simulink model "FOC"  (R2015b)
settings: Solver=VariableStepAuto  StartTime=0.0  StopTime=1  FixedStep=1e-5  RelTol=1e-3
model workspace (MAT data in the model file):
  J = 0.02
  Lm = 0.651
  Lr = 0.671
  Ls = 0.666
  P = 4
  Rr = 3.24
  Rs = 4.25
  theta0 = 0
undefined symbols (not defined in the file or in its folder): magnitude
libraries: powerlib x13, simulink x3
settings Model: Creator=yoush  LastModifiedBy=yoush

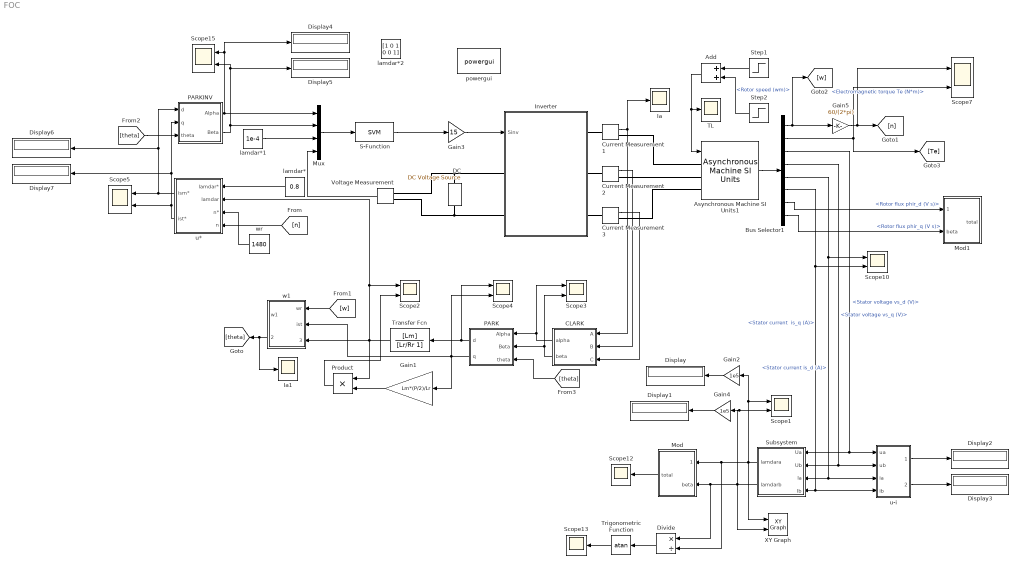
== system FOC ==
  Add : Sum
  Asynchronous Machine SI Units1 : powerlib/Machines/Asynchronous Machine SI Units  RotorType=Squirrel-cage  PresetModel=No  MechanicalLoad=Torque Tm  ShowDetailedParameters=on  ReferenceFrame=Stationary  Units=SI  MeasurementBus=off  NominalParameters=[20000 500 50]  Stator=[4.25 0.015]  Rotor=[3.24 0.020]  Cage1=[0.4155 0.002066]  Cage2=[0.4168 0.0003495]  Lm=0.651  Mechanical=[0.02 0 2]  PolePairs=2  InitialConditions=[ 1 0 0 0 0 0 0 0]  SimulateSaturation=off  Saturation=[14.03593122, 27.81365428, 53.79336849, 72.68890987, 97.98006896, 148.6815601, 215.7428561, 302.9841135, 428.7778367 ; 230, 322, 414, 460, 506, 552, 598, 644, 690]  LoadFlowParameters=1492000  TsPowergui=0  TsBlock=-1  IterativeModel=Trapezoidal non iterative  Pmec=1.492e+006
  Bus Selector1 : BusSelector  OutputSignals="Mechanical.Rotor speed (wm),Mechanical.Electromagnetic torque Te (N*m),Stator measurements.Stator voltage vs_d (V),Stator measurements.Stator voltage vs_q (V),Stator measurements.Stator current is_d (A),Stator measurements.Stator current  is_q (A),Rotor measurements.Rotor flux phir_d (V s),Rotor measurements.Rotor flux phir_q (V s)"
  CLARK : Subsystem
  Current Measurement1 : powerlib/Measurements/Current Measurement  PhasorSimulation=off  OutputType=Complex  PSBequivalent=0
  Current Measurement2 : powerlib/Measurements/Current Measurement  PhasorSimulation=off  OutputType=Complex  PSBequivalent=0
  Current Measurement3 : powerlib/Measurements/Current Measurement  PhasorSimulation=off  OutputType=Complex  PSBequivalent=0
  DC : powerlib/Electrical Sources/DC Voltage Source  Amplitude=500  Measurements=None
  Display{,1..7} (8 alike) : Display
  Divide : Product  Inputs=*/
  Gain1 : Gain  Gain=Lm*(P/2)/Lr
  Gain2 : Gain  Gain=1e5
  Gain3 : Gain  Gain=15
  Gain4 : Gain  Gain=1e5
  Gain5 : Gain  Gain=60/(2*pi)
  Ia : Scope
  Ia1 : Scope
  Inverter : Subsystem
  Mod : Subsystem
  Mod1 : Subsystem
  Mux : Mux
  PARK : Subsystem
  PARKINV : Subsystem
  Product : Product
  S-Function : S-Function  FunctionName=SVM  SFunctionDeploymentMode=off  EnableBusSupport=off
  Scope{1..5,7,10,15} (8 alike) : Scope  NumInputPorts=2
  Scope12 : Scope
  Scope13 : Scope
  Step1 : Step  Time=0.5  After=5  SampleTime=0
  Step2 : Step  Time=0.7  After=2  SampleTime=0
  Subsystem : Subsystem
  TL : Scope
  Transfer Fcn : TransferFcn  Numerator=[Lm]  Denominator=[Lr/Rr 1]
  Trigonometric Function : Trigonometry  Operator=atan
  Voltage Measurement : powerlib/Measurements/Voltage Measurement  PhasorSimulation=off  OutputType=Complex  PSBequivalent=0
  XY Graph : simulink/Sinks/XY Graph  xmin=-2  xmax=2  ymin=-2  ymax=2  st=-1
  lamdar* : Constant  Value=0.8
  lamdar*1 : Constant  Value=1e-4
  lamdar*2 : Constant  Value=[1 0 1 0 0 1]
  powergui : powerlib/powergui  Priority=1  SimulationMode=Discrete  SolverType=Tustin/Backward Euler (TBE)  SampleTime=1e-5  frequency=60  SPID=off  DisableSnubberDevices=off  DisableRonSwitches=off  DisableVfSwitches=off  SwTol=0  DisplayEquations=off  Interpol=off  ExternalGateDelay=off  methode=off  Ts=10  FunctionMessages=off  echomessages=off  HookPort=off  EnableUseOfTLC=off  x0status=blocks  frequencyindice=50  Pbase=100e6  ErrMax=1e-4  Iterations=50  UnitsV=kV  UnitsW=MW  buscounter=0  RestoreLinks=warning  ResistiveCurrentMeasurement=off  Frange=[0:2:500]  Ylog=off  Xlog=on  ShowGrid=off  save=off  variable=ZData  structure=we  ZoomFFT=off  StartTime=0.4  cycles=5  DisplayStyle=2  fundamental=100  FreqAxis=off  MaxFrequency=1000  frequencyindicesteady=1  RmsSteady=1  display=off
  u* : Subsystem
  u-i : Subsystem
  w1 : Subsystem
  wr : Constant  Value=1480
  wires:
  Current Measurement1/1 -> CLARK/1(A), Ia/1
  Add/1 -> Asynchronous Machine SI Units1/1, TL/1
  Step1/1 -> Add/1
  Step2/1 -> Add/2
  Asynchronous Machine SI Units1/1 -> Bus Selector1/1
  Bus Selector1/1 -> Gain5/1, [w]  "<Rotor speed (wm)>"
  Gain5/1 -> Scope7/1, [n]
  Bus Selector1/2 -> Scope7/2, [Te]  "<Electromagnetic torque Te (N*m)>"
  Current Measurement2/1 -> CLARK/2(B)
  Current Measurement3/1 -> CLARK/3(C)
  CLARK/1(alpha) -> Scope3/1, PARK/1(Alpha)
  CLARK/2(beta) -> Scope3/2, PARK/2(Beta)
  Subsystem/1(lamdara) -> Gain2/1, Scope1/1, XY Graph/1, Divide/2, Mod/1(alpha)
  Subsystem/2(lamdarb) -> Gain4/1, Scope1/2, XY Graph/2, Divide/1, Mod/2(beta)
  PARK/2(q) -> Gain1/1, w1/2(ist), Scope4/2
  [n] -> u*/4(n)
  Gain3/1 -> Inverter/1(Sinv)
  lamdar*/1 -> u*/1(lamdar*)
  wr/1 -> u*/3(n*)
  PARK/1(d) -> Transfer Fcn/1, Scope4/1
  Bus Selector1/3 -> u-i/1(ua), Subsystem/1(Ua)  "<Stator voltage vs_d (V)>"
  Bus Selector1/4 -> u-i/2(ub), Subsystem/2(Ub)  "<Stator voltage vs_q (V)>"
  Bus Selector1/5 -> Scope10/1, u-i/3(ia), Subsystem/3(Ia)  "<Stator current is_d (A)>"
  Bus Selector1/6 -> u-i/4(ib), Subsystem/4(Ib), Scope10/2  "<Stator current  is_q (A)>"
  PARKINV/1(Alpha) -> Display4/1, Scope15/1, Mux/1
  PARKINV/2(Beta) -> Mux/2, Display5/1, Scope15/2
  Transfer Fcn/1 -> Product/1, u*/2(lamdar), Scope2/1, w1/3(lamdar)
  [w] -> w1/1(wr)
  Gain1/1 -> Product/2
  [theta] -> PARKINV/3(theta)
  Mod/1(total) -> Scope12/1
  Divide/1 -> Trigonometric Function/1
  Trigonometric Function/1 -> Scope13/1
  [theta] -> PARK/3(theta)
  Bus Selector1/7 -> Mod1/1(alpha)  "<Rotor flux phir_d (V s)>"
  Bus Selector1/8 -> Mod1/2(beta)  "<Rotor flux phir_q (V s)>"
  w1/2(theta) -> Ia1/1, [theta]
  u*/1(ism*) -> Scope5/1, Display6/1, PARKINV/1(d)
  u*/2(ist*) -> Scope5/2, PARKINV/2(q), Display7/1
  Product/1 -> Scope2/2
  Mux/1 -> S-Function/1
  lamdar*1/1 -> Mux/3
  Voltage Measurement/1 -> Mux/4
  Gain2/1 -> Display/1
  Gain4/1 -> Display1/1
  u-i/1(lamdaSA) -> Display2/1
  u-i/2(lamdaSB) -> Display3/1
  S-Function/1 -> Gain3/1
  connections:
  Inverter/RConn1 -- Current Measurement1/LConn1
  Inverter/RConn2 -- Current Measurement2/LConn1
  Inverter/RConn3 -- Current Measurement3/LConn1
  Asynchronous Machine SI Units1/LConn1 -- Current Measurement1/RConn1
  Asynchronous Machine SI Units1/LConn2 -- Current Measurement2/RConn1
  Asynchronous Machine SI Units1/LConn3 -- Current Measurement3/RConn1
  DC/RConn1 -- Inverter/LConn1 -- Voltage Measurement/LConn1
  DC/LConn1 -- Inverter/LConn2 -- Voltage Measurement/LConn2

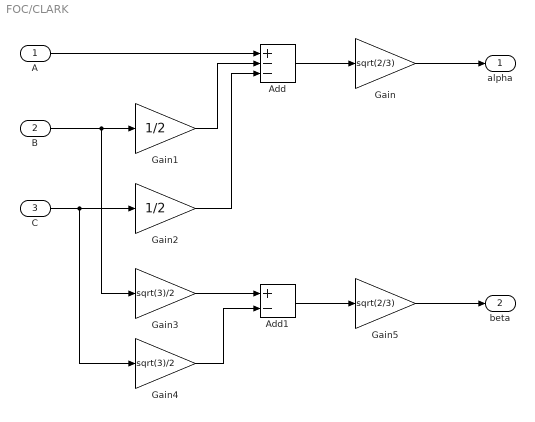
== system FOC/CLARK ==
  A : Inport
  B : Inport  Port=2
  C : Inport  Port=3
  Add : Sum  Inputs=+--
  Add1 : Sum  Inputs=+-
  Gain : Gain  Gain=sqrt(2/3)
  Gain1 : Gain  Gain=1/2
  Gain2 : Gain  Gain=1/2
  Gain3 : Gain  Gain=sqrt(3)/2
  Gain4 : Gain  Gain=sqrt(3)/2
  Gain5 : Gain  Gain=sqrt(2/3)
  alpha : Outport
  beta : Outport  Port=2
  wires:
  A/1 -> Add/1
  B/1 -> Gain3/1, Gain1/1
  Gain1/1 -> Add/2
  Gain2/1 -> Add/3
  C/1 -> Gain4/1, Gain2/1
  Gain3/1 -> Add1/1
  Gain4/1 -> Add1/2
  Add/1 -> Gain/1
  Add1/1 -> Gain5/1
  Gain/1 -> alpha/1
  Gain5/1 -> beta/1

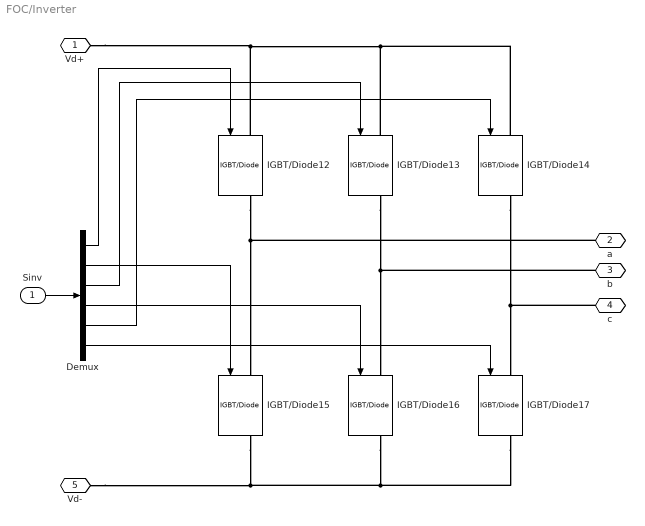
== system FOC/Inverter ==
  Sinv : Inport
  Demux : Demux  Outputs=6
  IGBT/Diode{12..17} (6 alike) : powerlib/Power Electronics/IGBT//Diode  Ron=1e-3  Rs=1e5  Cs=inf  Measurements=on
  Vd+ : PMIOPort  Port=1  Side=Left
  a : PMIOPort  Port=2  Side=Right
  b : PMIOPort  Port=3  Side=Right
  c : PMIOPort  Port=4  Side=Right
  Vd- : PMIOPort  Port=5  Side=Left
  wires:
  Demux/5 -> IGBT/Diode14/1
  Demux/4 -> IGBT/Diode16/1
  Demux/3 -> IGBT/Diode13/1
  Demux/6 -> IGBT/Diode17/1
  Demux/1 -> IGBT/Diode12/1
  Sinv/1 -> Demux/1
  Demux/2 -> IGBT/Diode15/1
  connections:
  IGBT/Diode12/RConn1 -- IGBT/Diode15/LConn1 -- a/RConn1
  IGBT/Diode13/RConn1 -- IGBT/Diode16/LConn1 -- b/RConn1
  IGBT/Diode14/RConn1 -- IGBT/Diode17/LConn1 -- c/RConn1
  IGBT/Diode17/RConn1 -- IGBT/Diode16/RConn1 -- Vd-/RConn1 -- IGBT/Diode15/RConn1
  IGBT/Diode12/LConn1 -- Vd+/RConn1 -- IGBT/Diode13/LConn1 -- IGBT/Diode14/LConn1

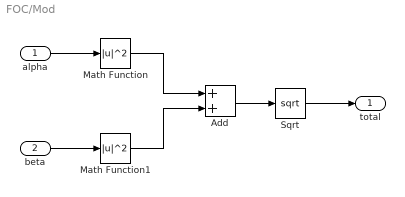
== system FOC/Mod ==
  alpha : Inport
  beta : Inport  Port=2
  Add : Sum
  Math Function : Math  Operator=magnitude^2  SaturateOnIntegerOverflow=on
  Math Function1 : Math  Operator=magnitude^2  SaturateOnIntegerOverflow=on
  Sqrt : Sqrt  SaturateOnIntegerOverflow=on
  total : Outport
  wires:
  alpha/1 -> Math Function/1
  beta/1 -> Math Function1/1
  Math Function/1 -> Add/1
  Math Function1/1 -> Add/2
  Add/1 -> Sqrt/1
  Sqrt/1 -> total/1

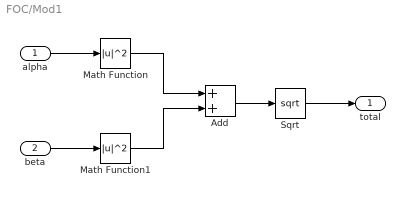
== system FOC/Mod1 ==
  alpha : Inport
  beta : Inport  Port=2
  Add : Sum
  Math Function : Math  Operator=magnitude^2  SaturateOnIntegerOverflow=on
  Math Function1 : Math  Operator=magnitude^2  SaturateOnIntegerOverflow=on
  Sqrt : Sqrt  SaturateOnIntegerOverflow=on
  total : Outport
  wires:
  alpha/1 -> Math Function/1
  beta/1 -> Math Function1/1
  Math Function/1 -> Add/1
  Math Function1/1 -> Add/2
  Add/1 -> Sqrt/1
  Sqrt/1 -> total/1

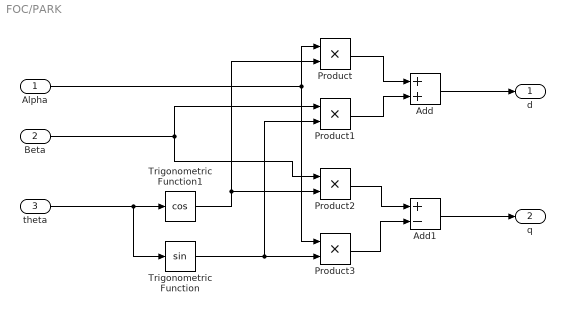
== system FOC/PARK ==
  Alpha : Inport
  Beta : Inport  Port=2
  theta : Inport  Port=3
  Add : Sum
  Add1 : Sum  Inputs=+-
  Product{,1..3} (4 alike) : Product
  Trigonometric Function : Trigonometry
  Trigonometric Function1 : Trigonometry  Operator=cos
  d : Outport
  q : Outport  Port=2
  wires:
  theta/1 -> Trigonometric Function1/1, Trigonometric Function/1
  Trigonometric Function1/1 -> Product/2, Product2/2
  Alpha/1 -> Product/1, Product3/1
  Trigonometric Function/1 -> Product1/2, Product3/2
  Beta/1 -> Product2/1, Product1/1
  Product/1 -> Add/1
  Product1/1 -> Add/2
  Add/1 -> d/1
  Product2/1 -> Add1/1
  Product3/1 -> Add1/2
  Add1/1 -> q/1

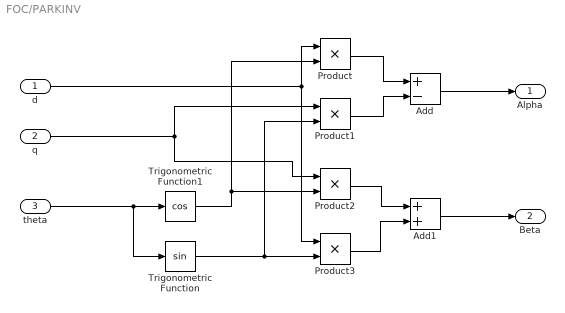
== system FOC/PARKINV ==
  d : Inport
  q : Inport  Port=2
  theta : Inport  Port=3
  Add : Sum  Inputs=+-
  Add1 : Sum
  Product{,1..3} (4 alike) : Product
  Trigonometric Function : Trigonometry
  Trigonometric Function1 : Trigonometry  Operator=cos
  Alpha : Outport
  Beta : Outport  Port=2
  wires:
  theta/1 -> Trigonometric Function1/1, Trigonometric Function/1
  Trigonometric Function1/1 -> Product/2, Product2/2
  d/1 -> Product/1, Product3/1
  Trigonometric Function/1 -> Product1/2, Product3/2
  q/1 -> Product2/1, Product1/1
  Product/1 -> Add/1
  Product1/1 -> Add/2
  Add/1 -> Alpha/1
  Product2/1 -> Add1/1
  Product3/1 -> Add1/2
  Add1/1 -> Beta/1

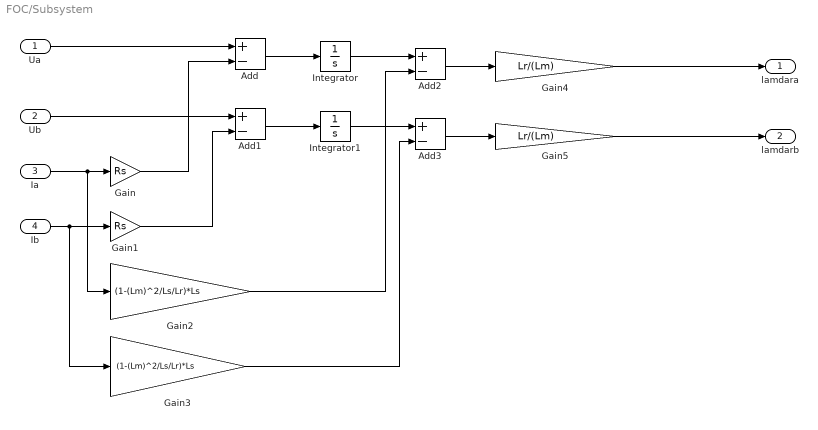
== system FOC/Subsystem ==
  Ua : Inport
  Ub : Inport  Port=2
  Ia : Inport  Port=3
  Ib : Inport  Port=4
  Add{,1..3} (4 alike) : Sum  Inputs=+-
  Gain : Gain  Gain=Rs
  Gain1 : Gain  Gain=Rs
  Gain2 : Gain  Gain=(1-(Lm)^2/Ls/Lr)*Ls
  Gain3 : Gain  Gain=(1-(Lm)^2/Ls/Lr)*Ls
  Gain4 : Gain  Gain=Lr/(Lm)
  Gain5 : Gain  Gain=Lr/(Lm)
  Integrator : Integrator
  Integrator1 : Integrator
  lamdara : Outport
  lamdarb : Outport  Port=2
  wires:
  Ib/1 -> Gain3/1, Gain1/1
  Ia/1 -> Gain2/1, Gain/1
  Ua/1 -> Add/1
  Gain/1 -> Add/2
  Ub/1 -> Add1/1
  Gain1/1 -> Add1/2
  Add/1 -> Integrator/1
  Add1/1 -> Integrator1/1
  Integrator/1 -> Add2/1
  Integrator1/1 -> Add3/1
  Gain2/1 -> Add2/2
  Gain3/1 -> Add3/2
  Add3/1 -> Gain5/1
  Add2/1 -> Gain4/1
  Gain4/1 -> lamdara/1
  Gain5/1 -> lamdarb/1

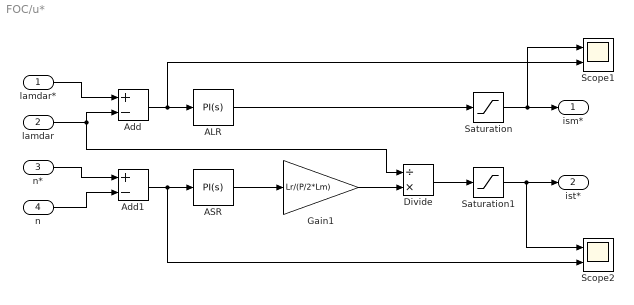
== system FOC/u* ==
  lamdar* : Inport
  lamdar : Inport  Port=2
  n* : Inport  Port=3
  n : Inport  Port=4
  ALR : simulink/Continuous/PID Controller  Controller=PI  TimeDomain=Continuous-time  SampleTime=-1  IntegratorMethod=Forward Euler  FilterMethod=Forward Euler  Form=Parallel  UseFilter=on  ControllerParametersSource=internal  P=2e2  I=0  D=0  N=100  InitialConditionSource=internal  InitialConditionForIntegrator=0  InitialConditionForFilter=0  ExternalReset=none  LimitOutput=off  UpperSaturationLimit=200  LowerSaturationLimit=-200  LinearizeAsGain=on  AntiWindupMode=none  Kb=1  TrackingMode=off  Kt=1  PParamMin=[]  PParamMax=[]  IParamMin=[]  IParamMax=[]  DParamMin=[]  DParamMax=[]  NParamMin=[]  NParamMax=[]  KbParamMin=[]  KbParamMax=[]  KtParamMin=[]  KtParamMax=[]  POutMin=[]  POutMax=[]  IOutMin=[]  IOutMax=[]  DOutMin=[]  DOutMax=[]  NOutMin=[]  NOutMax=[]  KbOutMin=[]  KbOutMax=[]  KtOutMin=[]  KtOutMax=[]  IntegratorOutMin=[]  IntegratorOutMax=[]  FilterOutMin=[]  FilterOutMax=[]  SumOutMin=[]  SumOutMax=[]  SumI1OutMin=[]  SumI1OutMax=[]  SumI2OutMin=[]  SumI2OutMax=[]  SumI3OutMin=[]  SumI3OutMax=[]  SumDOutMin=[]  SumDOutMax=[]  SaturationOutMin=[]  SaturationOutMax=[]  IntegratorContinuousStateAttributes=''  IntegratorStateMustResolveToSignalObject=off  IntegratorRTWStateStorageClass=Auto  FilterContinuousStateAttributes=''  FilterStateMustResolveToSignalObject=off  FilterRTWStateStorageClass=Auto  DifferentiatorICPrevScaledInput=0  DifferentiatorOutMin=[]  DifferentiatorOutMax=[]
  ASR : simulink/Continuous/PID Controller  Controller=PI  TimeDomain=Continuous-time  SampleTime=-1  IntegratorMethod=Forward Euler  FilterMethod=Forward Euler  Form=Parallel  UseFilter=on  ControllerParametersSource=internal  P=100  I=0  D=0  N=100  InitialConditionSource=internal  InitialConditionForIntegrator=0  InitialConditionForFilter=0  ExternalReset=none  LimitOutput=off  UpperSaturationLimit=1000  LowerSaturationLimit=-1000  LinearizeAsGain=on  AntiWindupMode=none  Kb=1  TrackingMode=off  Kt=1  PParamMin=[]  PParamMax=[]  IParamMin=[]  IParamMax=[]  DParamMin=[]  DParamMax=[]  NParamMin=[]  NParamMax=[]  KbParamMin=[]  KbParamMax=[]  KtParamMin=[]  KtParamMax=[]  POutMin=[]  POutMax=[]  IOutMin=[]  IOutMax=[]  DOutMin=[]  DOutMax=[]  NOutMin=[]  NOutMax=[]  KbOutMin=[]  KbOutMax=[]  KtOutMin=[]  KtOutMax=[]  IntegratorOutMin=[]  IntegratorOutMax=[]  FilterOutMin=[]  FilterOutMax=[]  SumOutMin=[]  SumOutMax=[]  SumI1OutMin=[]  SumI1OutMax=[]  SumI2OutMin=[]  SumI2OutMax=[]  SumI3OutMin=[]  SumI3OutMax=[]  SumDOutMin=[]  SumDOutMax=[]  SaturationOutMin=[]  SaturationOutMax=[]  IntegratorContinuousStateAttributes=''  IntegratorStateMustResolveToSignalObject=off  IntegratorRTWStateStorageClass=Auto  FilterContinuousStateAttributes=''  FilterStateMustResolveToSignalObject=off  FilterRTWStateStorageClass=Auto  DifferentiatorICPrevScaledInput=0  DifferentiatorOutMin=[]  DifferentiatorOutMax=[]
  Add : Sum  Inputs=+-
  Add1 : Sum  Inputs=+-
  Divide : Product  Inputs=/*
  Gain1 : Gain  Gain=Lr/(P/2*Lm)
  Saturation : Saturate  UpperLimit=1000  LowerLimit=-1000
  Saturation1 : Saturate  UpperLimit=1000  LowerLimit=-1000
  Scope1 : Scope  NumInputPorts=2
  Scope2 : Scope  NumInputPorts=2
  ism* : Outport
  ist* : Outport  Port=2
  wires:
  lamdar*/1 -> Add/1
  lamdar/1 -> Divide/1, Add/2
  n*/1 -> Add1/1
  n/1 -> Add1/2
  Add/1 -> Scope1/2, ALR/1
  Add1/1 -> Scope2/2, ASR/1
  ALR/1 -> Saturation/1
  ASR/1 -> Gain1/1
  Gain1/1 -> Divide/2
  Divide/1 -> Saturation1/1
  Saturation/1 -> Scope1/1, ism*/1
  Saturation1/1 -> Scope2/1, ist*/1

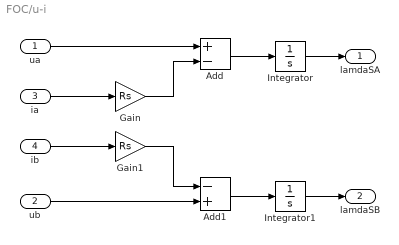
== system FOC/u-i ==
  ua : Inport
  ub : Inport  Port=2
  ia : Inport  Port=3
  ib : Inport  Port=4
  Add : Sum  Inputs=+-
  Add1 : Sum  Inputs=-+
  Gain : Gain  Gain=Rs
  Gain1 : Gain  Gain=Rs
  Integrator : Integrator
  Integrator1 : Integrator
  lamdaSA : Outport
  lamdaSB : Outport  Port=2
  wires:
  ib/1 -> Gain1/1
  ia/1 -> Gain/1
  Gain/1 -> Add/2
  ua/1 -> Add/1
  ub/1 -> Add1/2
  Gain1/1 -> Add1/1
  Add/1 -> Integrator/1
  Add1/1 -> Integrator1/1
  Integrator1/1 -> lamdaSB/1
  Integrator/1 -> lamdaSA/1

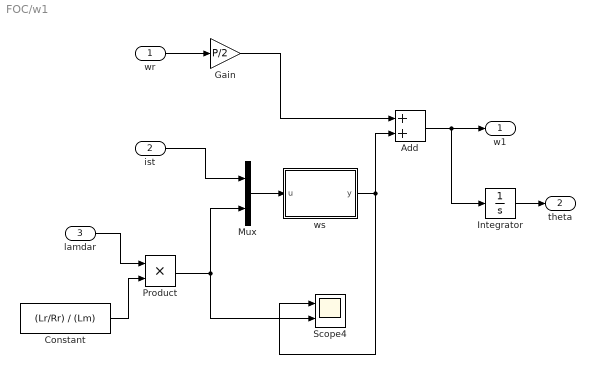
== system FOC/w1 ==
  wr : Inport
  ist : Inport  Port=2
  lamdar : Inport  Port=3
  Add : Sum
  Constant : Constant  Value=(Lr/Rr) / (Lm)
  Gain : Gain  Gain=P/2
  Integrator : Integrator
  Mux : Mux  Inputs=2
  Product : Product
  Scope4 : Scope  NumInputPorts=2
  ws : MATLAB Function  TreatAsAtomicUnit=on
  w1 : Outport
  theta : Outport  Port=2
  wires:
  ist/1 -> Mux/1
  Mux/1 -> ws/1(u)
  ws/1(y) -> Scope4/1, Add/2
  wr/1 -> Gain/1
  Add/1 -> Integrator/1, w1/1
  Gain/1 -> Add/1
  lamdar/1 -> Product/1
  Constant/1 -> Product/2
  Product/1 -> Mux/2, Scope4/2
  Integrator/1 -> theta/1

== matlab function FOC/w1/ws ==
  data: u input; y output
function y = fcn(u)
if (u(2) > 1e-6)
    y = u(1) / u(2);
else
    y = 0;
end
